simulink library "PC_Simulator_Lib"  (Simulink 8.2)
settings: Solver=ode45  StartTime=0.0  StopTime=10.0  RelTol=1e-3
values from neighbouring files (symbols this model uses):
  data = [r1 r2 r3 r4 L1 L2 L3 L4]    [strasse_Bedatung_HNI_ITI.m]
  distSameLane = 60    [InitialisationsEnv.m]
  eng_speed = [0 60 120 180 240 300 360 420 480 540 600 660 ... (101 elements, 1x101)]    [engine_table.mat]    (also in motor_parameter_calc.m = omega)
  Heading_init = 0    [Start.m]
  inertiaLateral = 25*(radiusWheel)^2    (= 4.129024)    [Start.m]
  laneWidth = 3.6    [InitialisationsEnv.m]    (also in strasse_Bedatung_HNI_ITI.m)
  omega_engine = [0.000000 150.000000 500.000000 1000.000000 1500.000000 2000.000000 2500.000000 3000.000000 3500.000000 4000.000000 4500.000000 5000.000000 5500.000000 6000.000000]    [friction_tables.m]
  omega_max = 6000    [engine_table.mat]    (also in motor_parameter_calc.m)
  omega_wheel = [0 20 40 60 80 100 122 143.7 164]    [friction_tables.m]
  para_Fellow_8_Points = ADAS.Fellow_8_Points    [ADAS_parameters.m]
  position_start_x = [x1 x2 x3 x4 x5 x6 x7]    [strasse_Bedatung_HNI_ITI.m]
  position_start_y = [y1 y2 y3 y4 y5 y6 y7]    [strasse_Bedatung_HNI_ITI.m]
  rad3rdLine = 57.2    [InitialisationsEnv.m]    (also in strasse_Bedatung_HNI_ITI.m)
  radiusWheel = 16*2.54/100    (= 0.4064)    [Start.m]
  s_values = [S1 S2 S3 S4 S5 S6 S7]    [strasse_Bedatung_HNI_ITI.m]
  segmentLimits = [segment1EndThirdLine                   segment2EndThirdLine                   segment3EndThirdLine                   segment4EndThirdLine                   segment5EndThirdLine                   segment6EndThirdLine                   segment7EndThirdLine                   segment8EndThirdLine                   ]    [InitialisationsEnv.m]    (also in strasse_Bedatung_HNI_ITI.m)
  setPosT = [-1.8 -5.4 -1.8 -5.4 -1.8 -5.4 -1.8 -5.4 -1.8 -5.4]    [InitialisationsEnv.m]
  torque = [297.089227105 300.997600937 304.800343044 308.497453426 312.088932082 315.574779014 318.95499422 322.229577701 325.398529457 328.461849487 331.419537793 334.271594373 ... (101 elements, 1x101)]    [engine_table.mat]    (also in motor_parameter_calc.m = g)
  Torque_lost = [0.000000 -8.777780 -15.000000 -26.800000 -29.600000 -32.700000 -35.900000 -39.300000 -42.800000 -46.500000 -50.300000 -54.300000 -58.500000 -62.800000 ]*0.6    [friction_tables.m]
  Torque_lost_wheel = [0.8 0.8 0.75 0.7 0.4 0.3 0.2 0.07 0.07]*0.2    [friction_tables.m]
  X_init = 0    [Start.m]
  Y_init = 1.8    [Start.m]
  Z_init = 0    [Start.m]
undefined symbols (not defined in the file or in its folder): Acc_Pedal, ADAS, Brake_Pedal, Joystick, Newton, Para, Raphson, Standard_Devices, Steering_Wheel_Angle, UDP_Protocol
libraries: simulink x43, rtwinlib x7, dspnetwork x2, simulink_extras x1, vrlib x1
(part 12 of 13)

== matlab function Drive_Train/4_Wheels_drive_train_and_Brake/RL/Fy_calculator ==
  data: lambda input double; Fy output double; alpha input double; V_x input double; Fz input double; mue input double

function Fy = FM_Fy(lambda,alpha,V_x,Fz,mue)
% This block supports an embeddable subset of the MATLAB language.
% See the help menu for details. 
%% Querkraft

kappa=lambda;
a=tan(alpha*pi/180);
%if V_x >=0 
 %   sign=1;
%else
 %   sign=-1;
%end
a_star=tan(alpha*pi/180)*sign(V_x);
F_z=Fz;
%Parameter

p_Cy1=1.193;
p_Ey1=-1.003;
p_Ey2=-0.532;
p_Ey3=-0.083;
p_Ey4=-4.787;
p_Ey5=0;
p_Ky1=14.95;
p_Ky2=2.13;
p_Ky3=-0.028;
p_Ky4=2;
p_Ky5=0;
p_Ky6=2.5;
p_Ky7=0;
p_Hy1=0;
p_Hy2=0;
p_Vy1=0;
p_Vy2=0;
p_Vy3=0;
p_Vy4=0;
r_By1=6.461;
r_By2=4.196;
r_By3=-0.015;
r_Cy1=1.081;
r_Ey1=0;
r_Ey2=0;
r_Hy1=0;
r_Hy2=0;
r_Vy1=0;
r_Vy2=0;
r_Vy3=0;
r_Vy4=0;
r_Vy5=0;
r_Vy6=0;

lambda_ykappa=1;
lambda_Fz0=1;
lambda_Kya=1;
lambda_Cy=1;
lambda_Vy=1;
lambda_muey=1;
lambda_Hy=1;
lambda_Kygamma=1;
lambda_Ey=1;
lambda_Vykappa=1;

% Unter der Annahme, dass die Vertikallast unverändert bleibt:
df_z=0;

%F_z=5500;
%mue=0.7;
chi_0=1;
chi_1=1;
chi_2=1;
chi_3=1;
chi_4=1;

% Annamhe, dass der Sturz bei null bleibt;

gamma=0;

% Berechnung

B_ykappa=(r_By1+r_By3*gamma^2)*cos(atan(r_By2*(a_star-r_By3)))*lambda_ykappa;
C_ykappa=r_Cy1;
E_ykappa=r_Ey1+r_Ey2*df_z;

S_Hykappa=r_Hy1+r_Hy2*df_z;
kappa_S=kappa+S_Hykappa;

G_ykappa0=cos(C_ykappa*atan(B_ykappa*S_Hykappa-E_ykappa*(B_ykappa*S_Hykappa-atan(B_ykappa*S_Hykappa))));
G_ykappa=cos(C_ykappa*atan(B_ykappa*kappa_S-E_ykappa*(B_ykappa*kappa_S-atan(B_ykappa*kappa_S))))/G_ykappa0;
% G_ykappa=cos(C_ykappa*atan(B_ykappa.*kappa_S-E_ykappa*(B_ykappa.*kappa_S-atan(B_ykappa.*kappa_S))))/G_ykappa0;















K_ygamma0=F_z*(p_Ky6+p_Ky7*df_z)*lambda_Kygamma;
S_Vygamma=F_z*(p_Vy3+p_Vy4*df_z)*gamma*lambda_Kygamma*lambda_muey*chi_2;
K_ya=p_Ky1*lambda_Fz0*F_z*sin(p_Ky4*atan(F_z/((p_Ky2+p_Ky5*gamma^2)*lambda_Fz0*F_z)))/(1+p_Ky3*gamma^2)*chi_3*lambda_Kya;
S_Vy=F_z*(p_Vy1+p_Vy2*df_z)*lambda_Vy*lambda_muey*chi_2+S_Vygamma;
S_Hy=(p_Hy1+p_Hy2*df_z)*lambda_Hy+(K_ygamma0*gamma-S_Vygamma)*chi_0/(K_ya+eps)+chi_4-1;

a_y=a+S_Hy;

D_Vykappa=mue*F_z*(r_Vy1+r_Vy2*df_z+r_Vy3*gamma)*cos(atan(r_Vy4*a))*chi_2;
S_Vykappa=D_Vykappa*sin(r_Vy5*atan(r_Vy6*kappa))*lambda_Vykappa;

C_y=p_Cy1*lambda_Cy;
D_y=mue*F_z*chi_2;
B_y=K_ya/(C_y*D_y+eps);
E_y=(p_Ey1+p_Ey2*df_z)*(1+p_Ey5*gamma^2-(p_Ey3+p_Ey4*gamma)*sign(a_y))*lambda_Ey;

F_y0=D_y*sin(C_y*atan(B_y*a_y-E_y*(B_y*a_y-atan(B_y*a_y))))+S_Vy;

F_y=G_ykappa*F_y0+S_Vykappa;

Fy=F_y;

== matlab function Drive_Train/4_Wheels_drive_train_and_Brake/RR/Fx_calculator ==
  data: lambda input double; Fx output double; alpha input double; Fz input double; mue input double
 function Fx = FM_Fx(lambda,alpha,Fz,mue)
% This block supports an embeddable subset of the MATLAB language.
% See the help menu for details. 

%% Längstkraft
kappa=lambda;
a=tan(alpha*pi/180);
F_z=Fz;
% Parameter
p_Cx1=1.685;
p_Ex1=0.344;
p_Ex2=0.095;
p_Ex3=-0.02;
p_Ex4=0;
p_Kx1=21.51;
p_Kx2=-0.163;
p_Kx3=0.245;
p_Hx1=0;
p_Hx2=0;
p_Vx1=0;
p_Vx2=0;
r_Cx1=1.0902;
r_Bx1=12.35;
r_Bx2=-10.77;
r_Bx3=0;
r_Ex1=0;
r_Ex2=0;
r_Hx1=0.007;            %r_Hx1=0.007;
gamma=0;
lambda_xa=1;
lambda_Cx=1;
lambda_Ex=1;
lambda_Hx=1;
lambda_Vx=1;
lambda_Kxkappa=1;
% Unter der Annahme, dass die Vertikallast unverändert bleibt:
df_z=0;

%F_z=5500;
%mue=0.7;
chi_1=1;

% Berechnung:

B_xa=(r_Bx1+r_Bx3*gamma^2)*cos(atan(r_Bx2*kappa))*lambda_xa;
C_xa=r_Cx1;
E_xa=r_Ex1+r_Ex2*df_z;

S_Hxa=r_Hx1;
a_S=a+S_Hxa;

G_xa0=cos(C_xa*atan(B_xa*S_Hxa-E_xa*(B_xa*S_Hxa-atan(B_xa*S_Hxa))));
G_xa=cos(C_xa*atan(B_xa*a_S-E_xa*(B_xa*a_S-atan(B_xa*a_S))))/G_xa0;

K_xkappa=F_z*(p_Kx1+p_Kx2*df_z)*exp(p_Kx3*df_z)*lambda_Kxkappa;
C_x=p_Cx1*lambda_Cx;
D_x=mue*F_z*chi_1;
B_x=K_xkappa/(C_x*D_x+eps);
E_x=(p_Ex1+p_Ex2*df_z+p_Ex3*df_z^2)*(1-p_Ex4*sign(kappa))*lambda_Ex;

S_Vx=F_z*(p_Vx1+p_Vx2*df_z)*lambda_Vx*lambda_Hx*chi_1;
S_Hx=(p_Hx1+p_Hx2*df_z)*lambda_Hx;
kappa_x=kappa+S_Hx;

F_x0 = D_x*sin(C_x*atan(B_x*kappa_x-E_x*(B_x*kappa_x-atan(B_x*kappa_x))))+S_Vx;
% F_x0 = D_x*sin(C_x*atan(B_x*kappa_x-E_x.*(B_x*kappa_x-atan(B_x*kappa_x))))+S_Vx;
F_x = G_xa*F_x0;
% if F_x>249;
%     F_x=249;
% end
Fx=F_x;

== matlab function Drive_Train/4_Wheels_drive_train_and_Brake/RR/Fy_calculator ==
  data: lambda input double; Fy output double; alpha input double; V_x input double; Fz input double; mue input double

function Fy = FM_Fy(lambda,alpha,V_x,Fz,mue)
% This block supports an embeddable subset of the MATLAB language.
% See the help menu for details. 
%% Querkraft

kappa=lambda;
a=tan(alpha*pi/180);
%if V_x >=0 
 %   sign=1;
%else
 %   sign=-1;
%end
a_star=tan(alpha*pi/180)*sign(V_x);
F_z=Fz;
%Parameter

p_Cy1=1.193;
p_Ey1=-1.003;
p_Ey2=-0.532;
p_Ey3=-0.083;
p_Ey4=-4.787;
p_Ey5=0;
p_Ky1=14.95;
p_Ky2=2.13;
p_Ky3=-0.028;
p_Ky4=2;
p_Ky5=0;
p_Ky6=2.5;
p_Ky7=0;
p_Hy1=0;
p_Hy2=0;
p_Vy1=0;
p_Vy2=0;
p_Vy3=0;
p_Vy4=0;
r_By1=6.461;
r_By2=4.196;
r_By3=-0.015;
r_Cy1=1.081;
r_Ey1=0;
r_Ey2=0;
r_Hy1=0;
r_Hy2=0;
r_Vy1=0;
r_Vy2=0;
r_Vy3=0;
r_Vy4=0;
r_Vy5=0;
r_Vy6=0;

lambda_ykappa=1;
lambda_Fz0=1;
lambda_Kya=1;
lambda_Cy=1;
lambda_Vy=1;
lambda_muey=1;
lambda_Hy=1;
lambda_Kygamma=1;
lambda_Ey=1;
lambda_Vykappa=1;

% Unter der Annahme, dass die Vertikallast unverändert bleibt:
df_z=0;

%F_z=5500;
%mue=0.7;
chi_0=1;
chi_1=1;
chi_2=1;
chi_3=1;
chi_4=1;

% Annamhe, dass der Sturz bei null bleibt;

gamma=0;

% Berechnung

B_ykappa=(r_By1+r_By3*gamma^2)*cos(atan(r_By2*(a_star-r_By3)))*lambda_ykappa;
C_ykappa=r_Cy1;
E_ykappa=r_Ey1+r_Ey2*df_z;

S_Hykappa=r_Hy1+r_Hy2*df_z;
kappa_S=kappa+S_Hykappa;

G_ykappa0=cos(C_ykappa*atan(B_ykappa*S_Hykappa-E_ykappa*(B_ykappa*S_Hykappa-atan(B_ykappa*S_Hykappa))));
G_ykappa=cos(C_ykappa*atan(B_ykappa*kappa_S-E_ykappa*(B_ykappa*kappa_S-atan(B_ykappa*kappa_S))))/G_ykappa0;
% G_ykappa=cos(C_ykappa*atan(B_ykappa.*kappa_S-E_ykappa*(B_ykappa.*kappa_S-atan(B_ykappa.*kappa_S))))/G_ykappa0;















K_ygamma0=F_z*(p_Ky6+p_Ky7*df_z)*lambda_Kygamma;
S_Vygamma=F_z*(p_Vy3+p_Vy4*df_z)*gamma*lambda_Kygamma*lambda_muey*chi_2;
K_ya=p_Ky1*lambda_Fz0*F_z*sin(p_Ky4*atan(F_z/((p_Ky2+p_Ky5*gamma^2)*lambda_Fz0*F_z)))/(1+p_Ky3*gamma^2)*chi_3*lambda_Kya;
S_Vy=F_z*(p_Vy1+p_Vy2*df_z)*lambda_Vy*lambda_muey*chi_2+S_Vygamma;
S_Hy=(p_Hy1+p_Hy2*df_z)*lambda_Hy+(K_ygamma0*gamma-S_Vygamma)*chi_0/(K_ya+eps)+chi_4-1;

a_y=a+S_Hy;

D_Vykappa=mue*F_z*(r_Vy1+r_Vy2*df_z+r_Vy3*gamma)*cos(atan(r_Vy4*a))*chi_2;
S_Vykappa=D_Vykappa*sin(r_Vy5*atan(r_Vy6*kappa))*lambda_Vykappa;

C_y=p_Cy1*lambda_Cy;
D_y=mue*F_z*chi_2;
B_y=K_ya/(C_y*D_y+eps);
E_y=(p_Ey1+p_Ey2*df_z)*(1+p_Ey5*gamma^2-(p_Ey3+p_Ey4*gamma)*sign(a_y))*lambda_Ey;

F_y0=D_y*sin(C_y*atan(B_y*a_y-E_y*(B_y*a_y-atan(B_y*a_y))))+S_Vy;

F_y=G_ykappa*F_y0+S_Vykappa;

Fy=F_y;

== matlab function Drive_Train/4_Wheels_drive_train_and_Brake/FR/Fx_calculator ==
  data: lambda input double; Fx output double; alpha input double; Fz input double; mue input double
 function Fx = FM_Fx(lambda,alpha,Fz,mue)
% This block supports an embeddable subset of the MATLAB language.
% See the help menu for details. 

%% Längstkraft
kappa=lambda;
a=tan(alpha*pi/180);
F_z=Fz;
% Parameter
p_Cx1=1.685;
p_Ex1=0.344;
p_Ex2=0.095;
p_Ex3=-0.02;
p_Ex4=0;
p_Kx1=21.51;
p_Kx2=-0.163;
p_Kx3=0.245;
p_Hx1=0;
p_Hx2=0;
p_Vx1=0;
p_Vx2=0;
r_Cx1=1.0902;
r_Bx1=12.35;
r_Bx2=-10.77;
r_Bx3=0;
r_Ex1=0;
r_Ex2=0;
r_Hx1=0.007;            %r_Hx1=0.007;
gamma=0;
lambda_xa=1;
lambda_Cx=1;
lambda_Ex=1;
lambda_Hx=1;
lambda_Vx=1;
lambda_Kxkappa=1;
% Unter der Annahme, dass die Vertikallast unverändert bleibt:
df_z=0;

%F_z=5500;
%mue=0.7;
chi_1=1;

% Berechnung:

B_xa=(r_Bx1+r_Bx3*gamma^2)*cos(atan(r_Bx2*kappa))*lambda_xa;
C_xa=r_Cx1;
E_xa=r_Ex1+r_Ex2*df_z;

S_Hxa=r_Hx1;
a_S=a+S_Hxa;

G_xa0=cos(C_xa*atan(B_xa*S_Hxa-E_xa*(B_xa*S_Hxa-atan(B_xa*S_Hxa))));
G_xa=cos(C_xa*atan(B_xa*a_S-E_xa*(B_xa*a_S-atan(B_xa*a_S))))/G_xa0;

K_xkappa=F_z*(p_Kx1+p_Kx2*df_z)*exp(p_Kx3*df_z)*lambda_Kxkappa;
C_x=p_Cx1*lambda_Cx;
D_x=mue*F_z*chi_1;
B_x=K_xkappa/(C_x*D_x+eps);
E_x=(p_Ex1+p_Ex2*df_z+p_Ex3*df_z^2)*(1-p_Ex4*sign(kappa))*lambda_Ex;

S_Vx=F_z*(p_Vx1+p_Vx2*df_z)*lambda_Vx*lambda_Hx*chi_1;
S_Hx=(p_Hx1+p_Hx2*df_z)*lambda_Hx;
kappa_x=kappa+S_Hx;

F_x0 = D_x*sin(C_x*atan(B_x*kappa_x-E_x*(B_x*kappa_x-atan(B_x*kappa_x))))+S_Vx;
% F_x0 = D_x*sin(C_x*atan(B_x*kappa_x-E_x.*(B_x*kappa_x-atan(B_x*kappa_x))))+S_Vx;
F_x = G_xa*F_x0;
% if F_x>249;
%     F_x=249;
% end
Fx=F_x;

== matlab function Drive_Train/4_Wheels_drive_train_and_Brake/FR/Fy_calculator ==
  data: lambda input double; Fy output double; alpha input double; V_x input double; Fz input double; mue input double

function Fy = FM_Fy(lambda,alpha,V_x,Fz,mue)
% This block supports an embeddable subset of the MATLAB language.
% See the help menu for details. 
%% Querkraft

kappa=lambda;
a=tan(alpha*pi/180);
%if V_x >=0 
 %   sign=1;
%else
 %   sign=-1;
%end
a_star=tan(alpha*pi/180)*sign(V_x);
F_z=Fz;
%Parameter

p_Cy1=1.193;
p_Ey1=-1.003;
p_Ey2=-0.532;
p_Ey3=-0.083;
p_Ey4=-4.787;
p_Ey5=0;
p_Ky1=14.95;
p_Ky2=2.13;
p_Ky3=-0.028;
p_Ky4=2;
p_Ky5=0;
p_Ky6=2.5;
p_Ky7=0;
p_Hy1=0;
p_Hy2=0;
p_Vy1=0;
p_Vy2=0;
p_Vy3=0;
p_Vy4=0;
r_By1=6.461;
r_By2=4.196;
r_By3=-0.015;
r_Cy1=1.081;
r_Ey1=0;
r_Ey2=0;
r_Hy1=0;
r_Hy2=0;
r_Vy1=0;
r_Vy2=0;
r_Vy3=0;
r_Vy4=0;
r_Vy5=0;
r_Vy6=0;

lambda_ykappa=1;
lambda_Fz0=1;
lambda_Kya=1;
lambda_Cy=1;
lambda_Vy=1;
lambda_muey=1;
lambda_Hy=1;
lambda_Kygamma=1;
lambda_Ey=1;
lambda_Vykappa=1;

% Unter der Annahme, dass die Vertikallast unverändert bleibt:
df_z=0;

%F_z=5500;
%mue=0.7;
chi_0=1;
chi_1=1;
chi_2=1;
chi_3=1;
chi_4=1;

% Annamhe, dass der Sturz bei null bleibt;

gamma=0;

% Berechnung

B_ykappa=(r_By1+r_By3*gamma^2)*cos(atan(r_By2*(a_star-r_By3)))*lambda_ykappa;
C_ykappa=r_Cy1;
E_ykappa=r_Ey1+r_Ey2*df_z;

S_Hykappa=r_Hy1+r_Hy2*df_z;
kappa_S=kappa+S_Hykappa;

G_ykappa0=cos(C_ykappa*atan(B_ykappa*S_Hykappa-E_ykappa*(B_ykappa*S_Hykappa-atan(B_ykappa*S_Hykappa))));
G_ykappa=cos(C_ykappa*atan(B_ykappa*kappa_S-E_ykappa*(B_ykappa*kappa_S-atan(B_ykappa*kappa_S))))/G_ykappa0;
% G_ykappa=cos(C_ykappa*atan(B_ykappa.*kappa_S-E_ykappa*(B_ykappa.*kappa_S-atan(B_ykappa.*kappa_S))))/G_ykappa0;















K_ygamma0=F_z*(p_Ky6+p_Ky7*df_z)*lambda_Kygamma;
S_Vygamma=F_z*(p_Vy3+p_Vy4*df_z)*gamma*lambda_Kygamma*lambda_muey*chi_2;
K_ya=p_Ky1*lambda_Fz0*F_z*sin(p_Ky4*atan(F_z/((p_Ky2+p_Ky5*gamma^2)*lambda_Fz0*F_z)))/(1+p_Ky3*gamma^2)*chi_3*lambda_Kya;
S_Vy=F_z*(p_Vy1+p_Vy2*df_z)*lambda_Vy*lambda_muey*chi_2+S_Vygamma;
S_Hy=(p_Hy1+p_Hy2*df_z)*lambda_Hy+(K_ygamma0*gamma-S_Vygamma)*chi_0/(K_ya+eps)+chi_4-1;

a_y=a+S_Hy;

D_Vykappa=mue*F_z*(r_Vy1+r_Vy2*df_z+r_Vy3*gamma)*cos(atan(r_Vy4*a))*chi_2;
S_Vykappa=D_Vykappa*sin(r_Vy5*atan(r_Vy6*kappa))*lambda_Vykappa;

C_y=p_Cy1*lambda_Cy;
D_y=mue*F_z*chi_2;
B_y=K_ya/(C_y*D_y+eps);
E_y=(p_Ey1+p_Ey2*df_z)*(1+p_Ey5*gamma^2-(p_Ey3+p_Ey4*gamma)*sign(a_y))*lambda_Ey;

F_y0=D_y*sin(C_y*atan(B_y*a_y-E_y*(B_y*a_y-atan(B_y*a_y))))+S_Vy;

F_y=G_ykappa*F_y0+S_Vykappa;

Fy=F_y;

== matlab function ADAS/Sensors_ADAS/Front_Long_Range_Radar_Sensor/First_STage_Coordinate_Transformation/Radar_Triangles_Transformation_From_Local2Global/Coord_Transformatin_Rotation1 ==
  data: roll input double; Trans_Local2Global output double; pitch input double; yaw input double
function Trans_Local2Global  = fcn(roll, pitch, yaw)


Trans_Local2Global=[ cos(pitch)*cos(yaw) cos(yaw)*sin(pitch)*sin(roll) - cos(roll)*sin(yaw) sin(roll)*sin(yaw) + cos(roll)*cos(yaw)*sin(pitch);
cos(pitch)*sin(yaw) cos(roll)*cos(yaw) + sin(pitch)*sin(roll)*sin(yaw) cos(roll)*sin(pitch)*sin(yaw) - cos(yaw)*sin(roll);
         -sin(pitch)                               cos(pitch)*sin(roll)                               cos(pitch)*cos(roll)];

== matlab function ADAS/Decision_Making_ADAS/Trajectory_calculatin_and_distance_control_and output_maping/Calculate_Desired_Trajectory/Road model ST_XY/st_xy ==
  data: x output double; s input double; t input double; y output double; z output double; headingAngle output double; curvature output double; friction output double; segmentNr output double; segmentLimits input double; laneWidth input double; rad3rdLine input double
function [x, y, z, headingAngle, curvature, friction, segmentNr]   = st_xy(s, t, segmentLimits, laneWidth, rad3rdLine)
%% Description
% This function transforms the (s,t) points of the road to (x,y) points
% From local coordinate system to global coordinate system
% s,t: s,t points of the local coordinate system in meters
% segmentLimits: Limits, i.e. ends, of road segments in meters
% laneWidth: The width of the lane in meter
% rad3rdLine: Radius of the third line, i.e lane marking, in meter  
% x,y: x,y points of the global coordinate system in meters
% headingAngle: Heading angle of the road at a specific road segment
% curvature: Curvature of the road at a specific road segment
% segmentNr: Segment number of a specific (s,t) point on the road
%% Simple schematic for a slice of the road
%     |          |         |          |          |
% FirstLine SecondLine ThirdLine FourthLine FifthLine 
%        Lane 2     Lane 1    Lane -1    Lane -2
%% Simple schematic for the road shape
%  _____________________
% (                     )
% |                     |
% |                     |
% |                     |
% (_____________________)

%% Initialise the outputs (Assign default values)
% Initialise x with zero
x = 0; 
% Initialise y with zero
y = 0;
% Initialise z with zero
z = 0;
% Initialise segmentNr with zero
segmentNr = 0;
% Initialise headingAngle with zero
headingAngle = 0;
% Initialise curvature with zero
curvature = 0;
% Initialise friction coefficient (Asphalt)
friction = 0.72;

%% Check (s,t) point against all segments
%% Check if the point is in the 1st road segment (Straight line)
if(s>=0)&&(s<segmentLimits(1))  
    % Calculate x component
    x = s;
    % Calculate y component
    y = t;
    % Calculate z value
    z = 0;
    % Calculate heading angle
    headingAngle = 0;
    % Calculate curvature
    curvature = 0;
    % Set friction value
    friction  = 0.72;
    % Set segment number
    segmentNr = 1;
%% Check if the point is in the 2nd road segment
elseif(s>=segmentLimits(1)) && (s<segmentLimits(2)) 
    % Calculate x component
    x = (rad3rdLine-t)*sin((s-segmentLimits(1))/rad3rdLine) + 600;
    % Calculate y component
    y = rad3rdLine - (rad3rdLine-t)*cos((s-segmentLimits(1))/rad3rdLine);
    % Calculate z value
    z = 0;
    % Calculate heading angle
    headingAngle = (180/pi)*(s-600)/rad3rdLine;
    % Calculate curvature
    curvature = 1/(rad3rdLine-t);
    % Set friction value
    friction  = 0.72;
    % Set segment number
    segmentNr = 2;
%% Check if the point is in the 3rd road segment  
elseif(s>=segmentLimits(2)) && (s<segmentLimits(3))
    % Calculate x component
    x = -t + 600 + rad3rdLine;
    % Calculate y component
    y = (s-segmentLimits(2)) + rad3rdLine;
    % Calculate z value
    z = 0;
    % Calculate heading angle
    headingAngle = 90;
    % Calculate curvature
    curvature = 0;
    % Set friction value
    friction  = 0.72;
    % Set segment number
    segmentNr = 3;
%% Check if the point is in the 4th road segment
elseif(s>=segmentLimits(3)) && (s<segmentLimits(4))
    % Calculate x component
    x = (rad3rdLine-t)*cos((s-segmentLimits(3))/rad3rdLine) - rad3rdLine + 600 + rad3rdLine;
    % Calculate y component
    y = (rad3rdLine-t)*sin((s-segmentLimits(3))/rad3rdLine) + 300 + rad3rdLine;
    % Calculate z value
    z = 0;
    % Calculate heading angle
    headingAngle = ((180/pi)*(s-(600+89.8857+300))/rad3rdLine) + 90;
    % Calculate curvature
    curvature = 1/(rad3rdLine-t);
    % Set friction value
    friction  = 0.72;
    % Set segment number
    segmentNr = 4;
%% Check if the point is in the 5th road segment
elseif(s>=segmentLimits(4))&&(s<segmentLimits(5))
    % Calculate x component
    x = -(s-segmentLimits(4)) + 600;
    % Calculate y component
    y = -t + (4*laneWidth) + 50 + 300 + 50;
    % Calculate z value
    z = 0;
    % Calculate heading angle
    headingAngle = 180;
    % Calculate curvature
    curvature = 0;
    % Set friction value
    friction  = 0.72;
    % Set segment number
    segmentNr = 5;
%% Check if the point is in the 6th road segment  
elseif(s>=segmentLimits(5))&&(s<segmentLimits(6))
    % Calculate x component
    x = -(rad3rdLine-t)*sin((s-segmentLimits(5))/rad3rdLine);
    % Calculate y component
    y = (rad3rdLine-t)*cos((s-segmentLimits(5))/rad3rdLine)- rad3rdLine + (4*laneWidth) + 50 + 300 + 50;
    % Calculate z value
    z = 0;
    % Calculate heading angle
    headingAngle = ((180/pi)*(s-(600+89.8857+300+89.8857+600))/rad3rdLine) + 180;
    % Calculate curvature
    curvature = 1/(rad3rdLine-t);
    % Set friction value
    friction  = 0.72;
    % Set segment number
    segmentNr = 6;
%% Check if the point is in the 7th road segment 
elseif(s>=segmentLimits(6))&&(s<segmentLimits(7))
    % Calculate x component
    x = t- 50 - 3.6 - 3.6;
    % Calculate y component
    y = -(s-segmentLimits(6)) + (2*laneWidth) + 300 + 50;
    % Calculate z value
    z = 0;
    % Calculate heading angle
    headingAngle = 270;
    % Calculate curvature
    curvature = 0;
    % Set friction value
    friction  = 0.72;
    % Set segment number
    segmentNr = 7;
%% Check if the point is in the 8th road segment 
elseif(s>=segmentLimits(7))&&(s<segmentLimits(8))
    % Calculate x component
    x = rad3rdLine-(rad3rdLine-t)*cos((s-segmentLimits(7))/rad3rdLine) - rad3rdLine;
    % Calculate y component
    y = -(rad3rdLine-t)*sin((s-segmentLimits(7))/rad3rdLine) + rad3rdLine; 
    % Calculate z value
    z = 0;
    % Calculate heading angle
    headingAngle = ((180/pi)*(s-(600+89.8857+300+89.8857+600+89.8857+300))/rad3rdLine) + 270;
    % Calculate curvature
    curvature = 1/(rad3rdLine-t);
    % Set friction value
    friction  = 0.72;
    % Set segment number
    segmentNr = 8;
end
end

== matlab function ADAS/Decision_Making_ADAS/Trajectory_calculatin_and_distance_control_and output_maping/Calculate_Desired_Trajectory/Strasse_xy/Embedded MATLAB Function ==
  data: data input double; position_start_x input double; position_start_y input double; s_values input double; x input double; y input double; z output double; psi output double; mue output double; s output double; t output double
function [z,psi,mue,s,t] = fcn(data,position_start_x,position_start_y,s_values,x,y)


breite=14.4;
margin=3;

if x>=0 && x<position_start_x(1) && y>=-(breite/2+margin) && y<=(breite/2+margin)                                               %S1
    s=x;
    t=y;
    psi=0;
else if x>=position_start_x(1) && x<(position_start_x(2)+breite/2+margin) && y>=-(breite/2+margin) && y<=position_start_y(2)    %S2
        phi=atan((x-position_start_x(1))/(position_start_y(2)-y));
        r=sqrt((x-position_start_x(1))^2 + (position_start_y(2)-y)^2);
        s=data(1)*phi+s_values(1);
        t=data(1)-r;
        psi=phi;
        
else if x>=(position_start_x(2)-breite/2-margin) && x<=(position_start_x(2)+breite/2+margin) && y>position_start_y(2) && y<position_start_y(3)  %S3
        s=s_values(2)+(y-position_start_y(2));
        t=position_start_x(2)-x;
        psi=pi/2;
        
else if  x<=(position_start_x(3)+breite/2+margin) && x>=(position_start_x(4)) && y>=position_start_y(3) && y<=(position_start_y(4)+breite/2+margin)   %S4
        phi=atan((y-position_start_y(3))/(x-position_start_x(4)));
        r=sqrt((y-position_start_y(3))^2+(x-position_start_x(4))^2);
        s=s_values(3)+data(2)*phi;
        t=data(2)-r;
        psi=pi/2+phi;
        
else if x<position_start_x(4) && x>position_start_x(5) && y>=(position_start_y(4)-breite/2-margin) && y<(position_start_y(4)+breite/2+margin)   %S5
        s=s_values(4)+(position_start_x(4)-x);
        t=position_start_y(4)-y;
        psi=pi;
        
else if x<=position_start_x(5) && x>=(position_start_x(6)-breite/2-margin) && y>=position_start_y(6) && y<=(position_start_y(5)+breite/2+margin)   %S6
        phi=atan(-x/(y-position_start_y(6)));
        r=sqrt((x)^2+(y-position_start_y(6))^2);
        s=s_values(5)+data(3)*phi;
        t=data(3)-r;
        psi=pi+phi;
        
else if x>=(position_start_x(6)-breite/2-margin) && x<=(position_start_x(6)+breite/2+margin) && y>position_start_y(7) && y<position_start_y(6)   %S7
        s=s_values(6)+(position_start_y(6)-y);
        t=x-position_start_x(6);
        psi=3*pi/2;
        
else if x>=(position_start_x(7)-breite/2-margin) && x<0 && y>=(-breite/2-margin) && y<=position_start_y(7)   %S8
        phi=atan((position_start_y(7)-y)/(-x));
        r=sqrt((position_start_y(7)-y)^2+(x)^2);
        s=s_values(7)+data(4)*phi;
        t=data(4)-r;
        psi=3*pi/2+phi;     
        

     else
         s=0;
         t=0;
         psi=0;

    end
    end
    end
    end
    end
    end
    end
end
    
z=0;
mue=1;

== matlab function ADAS/Sensors_ADAS/Front_Long_Range_Radar_Sensor/Coordinate_TRansformation_of_Fellows_Points_Plus_Calculation_Distances_And_Angles/MATLAB Function ==
  data: Objects_Dectected input double; Position_Fellows input double; Oriantation_Fellows input double; Apex_Pos_Global input double; yaw_VUT input double; delta_s output double; Angle output double; para_num_fellow parameter double; para_Fellow_8_Points parameter double; position output double
function [delta_s,Angle,position] = fcn(Objects_Dectected,Position_Fellows,Oriantation_Fellows,Apex_Pos_Global,yaw_VUT,para_num_fellow,para_Fellow_8_Points)
%%
Fellow_Points=zeros(para_num_fellow,24);
delta_distance=zeros(para_num_fellow,2);
Angles_Array=zeros(para_num_fellow,1);
position_Array=zeros(para_num_fellow,3,2);
% index=-1; %only for testing

% pass inputs and calculate the transformation matrix 
for i=0:para_num_fellow-1
    if Objects_Dectected(i+1)==1
    roll=Oriantation_Fellows(i*3+1);
    pitch=Oriantation_Fellows(i*3+2);
    yaw=Oriantation_Fellows(i*3+3);
    Trans_Local2Global=[ cos(pitch)*cos(yaw) cos(yaw)*sin(pitch)*sin(roll) - cos(roll)*sin(yaw) sin(roll)*sin(yaw) + cos(roll)*cos(yaw)*sin(pitch);
    cos(pitch)*sin(yaw) cos(roll)*cos(yaw) + sin(pitch)*sin(roll)*sin(yaw) cos(roll)*sin(pitch)*sin(yaw) - cos(yaw)*sin(roll);
         -sin(pitch)                               cos(pitch)*sin(roll)                               cos(pitch)*cos(roll)];
     
     FLU=Trans_Local2Global*para_Fellow_8_Points.FLU+[Position_Fellows(i*3+1);Position_Fellows(i*3+2);Position_Fellows(i*3+3)];
     FLL=Trans_Local2Global*para_Fellow_8_Points.FLL+[Position_Fellows(i*3+1);Position_Fellows(i*3+2);Position_Fellows(i*3+3)];
     FRU=Trans_Local2Global*para_Fellow_8_Points.FRU+[Position_Fellows(i*3+1);Position_Fellows(i*3+2);Position_Fellows(i*3+3)];
     FRL=Trans_Local2Global*para_Fellow_8_Points.FRL+[Position_Fellows(i*3+1);Position_Fellows(i*3+2);Position_Fellows(i*3+3)];
     RLU=Trans_Local2Global*para_Fellow_8_Points.RLU+[Position_Fellows(i*3+1);Position_Fellows(i*3+2);Position_Fellows(i*3+3)];
     RLL=Trans_Local2Global*para_Fellow_8_Points.RLL+[Position_Fellows(i*3+1);Position_Fellows(i*3+2);Position_Fellows(i*3+3)];
     RRU=Trans_Local2Global*para_Fellow_8_Points.RRU+[Position_Fellows(i*3+1);Position_Fellows(i*3+2);Position_Fellows(i*3+3)];
     RRL=Trans_Local2Global*para_Fellow_8_Points.RRL+[Position_Fellows(i*3+1);Position_Fellows(i*3+2);Position_Fellows(i*3+3)];
     A=[FLU ; FLL ; FRU ; FRL ; RLU ; RLL ; RRU ; RRL];
     Fellow_Points(i+1,:)=A;  %what is that
     dist1=sqrt(sum((Apex_Pos_Global-FLU).^2));
     dist2=sqrt(sum((Apex_Pos_Global-FLL).^2));
     dist3=sqrt(sum((Apex_Pos_Global-FRU).^2));
     dist4=sqrt(sum((Apex_Pos_Global-FRL).^2));
     dist5=sqrt(sum((Apex_Pos_Global-RLU).^2));
     dist6=sqrt(sum((Apex_Pos_Global-RLL).^2));
     dist7=sqrt(sum((Apex_Pos_Global-RRU).^2));
     dist8=sqrt(sum((Apex_Pos_Global-RRL).^2));     
     
     Dist=[dist1 dist2 dist3 dist4 dist5 dist6 dist7 dist8];
     [~, index_Sort_Arr]=sort(Dist);
     Angle1=abs((atan2((A((index_Sort_Arr(1)-1)*3+2)-Apex_Pos_Global(2)),(A((index_Sort_Arr(1)-1)*3+1)-Apex_Pos_Global(1))))-yaw_VUT);
     Angle2=abs((atan2((A((index_Sort_Arr(2)-1)*3+2)-Apex_Pos_Global(2)),(A((index_Sort_Arr(2)-1)*3+1)-Apex_Pos_Global(1))))-yaw_VUT);
     Angle3=abs((atan2((A((index_Sort_Arr(3)-1)*3+2)-Apex_Pos_Global(2)),(A((index_Sort_Arr(3)-1)*3+1)-Apex_Pos_Global(1))))-yaw_VUT);
     [~,index_angle_min]=min([Angle1 Angle2 Angle3]);
     [~,index_angle_max]=max([Angle1 Angle2 Angle3]);
     index_min=index_Sort_Arr(index_angle_min);
     index_max=index_Sort_Arr(index_angle_max);     
%      [delta_distance(i+1), index]=min([dist1 dist2 dist3 dist4 dist5 dist6 dist7 dist8]);
     delta_distance(i+1,1)=Dist(index_min);
     delta_distance(i+1,2)=Dist(index_max);
%      Angles_Array(i+1)=(atan2((A((index-1)*3+2)-Apex_Pos_Global(2)),(A((index-1)*3+1)-Apex_Pos_Global(1))))-yaw_VUT;
%      position_Array(i+1,:)=[A((index-1)*3+1) A((index-1)*3+2) A((index-1)*3+3)];
     position_Array(i+1,:,1)=[A((index_min-1)*3+1) A((index_min-1)*3+2) A((index_min-1)*3+3)];
     position_Array(i+1,:,2)=[A((index_max-1)*3+1) A((index_max-1)*3+2) A((index_max-1)*3+3)];
    end
end
%%
%pass the output

delta_s=delta_distance;
Angle=Angles_Array;
position=position_Array;

== matlab function ADAS/Sensors_ADAS/Front_Mid_Range_Radar_Sensor/First_STage_Coordinate_Transformation/Radar_Triangles_Transformation_From_Local2Global/Coord_Transformatin_Rotation1 ==
  data: roll input double; Trans_Local2Global output double; pitch input double; yaw input double
function Trans_Local2Global  = fcn(roll, pitch, yaw)


Trans_Local2Global=[ cos(pitch)*cos(yaw) cos(yaw)*sin(pitch)*sin(roll) - cos(roll)*sin(yaw) sin(roll)*sin(yaw) + cos(roll)*cos(yaw)*sin(pitch);
cos(pitch)*sin(yaw) cos(roll)*cos(yaw) + sin(pitch)*sin(roll)*sin(yaw) cos(roll)*sin(pitch)*sin(yaw) - cos(yaw)*sin(roll);
         -sin(pitch)                               cos(pitch)*sin(roll)                               cos(pitch)*cos(roll)];

== stateflow chart ADAS/Unser_Interface_ADAS/ACC_User_Interface/ACC_User_Control ==
  state ActiveSet
    en:
    Set_Speed=Velocity_VUT;
    Last_Set_Speed=Velocity_VUT;
    ACC_State=1;
    First_Set=0;
    state Default
    state Plus
      en:
      Last_Set_Speed=min(Last_Set_Speed+5/3.6, 200/3.6);
      Set_Speed=Last_Set_Speed;
    state Minus
      Last_Set_Speed=max(Last_Set_Speed-5/3.6,0);
      Set_Speed=Last_Set_Speed;
    (default) -> Default
    Default -> Plus [order 1] : Button_Plus
    Default -> Minus [order 2] : Button_Minus
    Minus -> Default
    Plus -> Default
  state ActiveResume
    en:
    Set_Speed=Last_Set_Speed;
    ACC_State=1;
    state Default1
    state Minus1
      Last_Set_Speed=max(Last_Set_Speed-5/3.6,0);
      Set_Speed=Last_Set_Speed;
    state Plus1
      en:
      Last_Set_Speed=min(Last_Set_Speed+5/3.6, 200/3.6);
      Set_Speed=Last_Set_Speed;
    (default) -> Default1
    Default1 -> Plus1 [order 1] : Button_Plus
    Default1 -> Minus1 [order 2] : Button_Minus
    Minus1 -> Default1
    Plus1 -> Default1
  state Standby
    ACC_State=0;
  state Standby1
    ACC_State=0;
  Standby1 -> ActiveResume [order 1] : [Gas_Pedal_User<=Gas_Pedal_ACC]
  Standby -> ActiveResume [order 2] : Button_Resume[Gearbox_State==1 && First_Set==0 && Enabled_Systems==0]
  Standby -> ActiveSet [order 1] : Button_Plus || Button_Minus   [Gearbox_State==1 && Enabled_Systems==0 ]
  ActiveSet -> Standby [order 2] : [ Gearbox_State!=1 || Brake_Pedal_User>Brake_Pedal_ACC ]
  ActiveSet -> Standby [order 1] : Button_Stop
  ActiveSet -> Standby1 [order 3] : [Gas_Pedal_User>Gas_Pedal_ACC]
  ActiveResume -> Standby1 [order 3] : [Gas_Pedal_User>Gas_Pedal_ACC]
  ActiveResume -> Standby [order 1] : Button_Stop
  ActiveResume -> Standby [order 2] : [ Gearbox_State!=1 || Brake_Pedal_User>Brake_Pedal_ACC ]
  (default) -> Standby
  Standby1 -> Standby [order 2] : Button_Stop
  Standby1 -> Standby [order 3] : [ Gearbox_State!=1 || Brake_Pedal_User>Brake_Pedal_ACC ]
  data: ACC_State output double =0; Gearbox_State input double; Gas_Pedal_User input double; Brake_Pedal_User input double; Velocity_VUT input double; Gas_Pedal_ACC input double; Brake_Pedal_ACC input double; Set_Speed output double =0; Last_Set_Speed local double =0; First_Set local double =1; Enabled_Systems input double
  events: update input EITHER_EDGE_EVENT; Button_Plus input RISING_EDGE_EVENT; Button_Minus input RISING_EDGE_EVENT; Button_Stop input RISING_EDGE_EVENT; Button_Resume input RISING_EDGE_EVENT

== stateflow chart ADAS/Unser_Interface_ADAS/ACC_User_Interface/Time_Gap_switching ==
  state Sporty
    en:
    Time_Gap=1;
  state Comfortable
    en:
    Time_Gap=2.3;
  state SemiComfortable
    en:
    Time_Gap=1.8;
  state SemiSporty
    en:
    Time_Gap=1.3;
  note: the values and the modes
      | are from the Audi A8 Prese
  Sporty -> SemiSporty : Button
  Comfortable -> Sporty : Button
  SemiSporty -> SemiComfortable : Button
  SemiComfortable -> Comfortable : Button
  (default) -> Comfortable
  data: Time_Gap output double
  events: Update input EITHER_EDGE_EVENT; Button input RISING_EDGE_EVENT

== stateflow chart ADAS/Unser_Interface_ADAS/Emergency_Brake/Emergency_brake_HMI_model ==
  state On
    en:
    State=1;
  state Off
    en:
    State=0;
  On -> Off : Button
  Off -> On : Button[Enabled_Systems==0]
  (default) -> Off
  data: State output double; Enabled_Systems input double
  events: Update input EITHER_EDGE_EVENT; Button input RISING_EDGE_EVENT

== matlab function ADAS/Sensors_ADAS/Front_Mid_Range_Radar_Sensor/Coordinate_TRansformation_of_Fellows_Points_Plus_Calculation_Distances_And_Angles/MATLAB Function ==
  data: Objects_Dectected input double; Position_Fellows input double; Oriantation_Fellows input double; Apex_Pos_Global input double; yaw_VUT input double; delta_s output double; Angle output double; para_num_fellow parameter double; para_Fellow_8_Points parameter double; position output double
function [delta_s,Angle,position] = fcn(Objects_Dectected,Position_Fellows,Oriantation_Fellows,Apex_Pos_Global,yaw_VUT,para_num_fellow,para_Fellow_8_Points)
%%
Fellow_Points=zeros(para_num_fellow,24);
delta_distance=zeros(para_num_fellow,2);
Angles_Array=zeros(para_num_fellow,1);
position_Array=zeros(para_num_fellow,3,2);
% index=-1; %only for testing

% pass inputs and calculate the transformation matrix 
for i=0:para_num_fellow-1
    if Objects_Dectected(i+1)==1
    roll=Oriantation_Fellows(i*3+1);
    pitch=Oriantation_Fellows(i*3+2);
    yaw=Oriantation_Fellows(i*3+3);
    Trans_Local2Global=[ cos(pitch)*cos(yaw) cos(yaw)*sin(pitch)*sin(roll) - cos(roll)*sin(yaw) sin(roll)*sin(yaw) + cos(roll)*cos(yaw)*sin(pitch);
    cos(pitch)*sin(yaw) cos(roll)*cos(yaw) + sin(pitch)*sin(roll)*sin(yaw) cos(roll)*sin(pitch)*sin(yaw) - cos(yaw)*sin(roll);
         -sin(pitch)                               cos(pitch)*sin(roll)                               cos(pitch)*cos(roll)];
     
     FLU=Trans_Local2Global*para_Fellow_8_Points.FLU+[Position_Fellows(i*3+1);Position_Fellows(i*3+2);Position_Fellows(i*3+3)];
     FLL=Trans_Local2Global*para_Fellow_8_Points.FLL+[Position_Fellows(i*3+1);Position_Fellows(i*3+2);Position_Fellows(i*3+3)];
     FRU=Trans_Local2Global*para_Fellow_8_Points.FRU+[Position_Fellows(i*3+1);Position_Fellows(i*3+2);Position_Fellows(i*3+3)];
     FRL=Trans_Local2Global*para_Fellow_8_Points.FRL+[Position_Fellows(i*3+1);Position_Fellows(i*3+2);Position_Fellows(i*3+3)];
     RLU=Trans_Local2Global*para_Fellow_8_Points.RLU+[Position_Fellows(i*3+1);Position_Fellows(i*3+2);Position_Fellows(i*3+3)];
     RLL=Trans_Local2Global*para_Fellow_8_Points.RLL+[Position_Fellows(i*3+1);Position_Fellows(i*3+2);Position_Fellows(i*3+3)];
     RRU=Trans_Local2Global*para_Fellow_8_Points.RRU+[Position_Fellows(i*3+1);Position_Fellows(i*3+2);Position_Fellows(i*3+3)];
     RRL=Trans_Local2Global*para_Fellow_8_Points.RRL+[Position_Fellows(i*3+1);Position_Fellows(i*3+2);Position_Fellows(i*3+3)];
     A=[FLU ; FLL ; FRU ; FRL ; RLU ; RLL ; RRU ; RRL];
     Fellow_Points(i+1,:)=A;  %what is that
     dist1=sqrt(sum((Apex_Pos_Global-FLU).^2));
     dist2=sqrt(sum((Apex_Pos_Global-FLL).^2));
     dist3=sqrt(sum((Apex_Pos_Global-FRU).^2));
     dist4=sqrt(sum((Apex_Pos_Global-FRL).^2));
     dist5=sqrt(sum((Apex_Pos_Global-RLU).^2));
     dist6=sqrt(sum((Apex_Pos_Global-RLL).^2));
     dist7=sqrt(sum((Apex_Pos_Global-RRU).^2));
     dist8=sqrt(sum((Apex_Pos_Global-RRL).^2));     
     
     Dist=[dist1 dist2 dist3 dist4 dist5 dist6 dist7 dist8];
     [~, index_Sort_Arr]=sort(Dist);
     Angle1=abs((atan2((A((index_Sort_Arr(1)-1)*3+2)-Apex_Pos_Global(2)),(A((index_Sort_Arr(1)-1)*3+1)-Apex_Pos_Global(1))))-yaw_VUT);
     Angle2=abs((atan2((A((index_Sort_Arr(2)-1)*3+2)-Apex_Pos_Global(2)),(A((index_Sort_Arr(2)-1)*3+1)-Apex_Pos_Global(1))))-yaw_VUT);
     Angle3=abs((atan2((A((index_Sort_Arr(3)-1)*3+2)-Apex_Pos_Global(2)),(A((index_Sort_Arr(3)-1)*3+1)-Apex_Pos_Global(1))))-yaw_VUT);
     [~,index_angle_min]=min([Angle1 Angle2 Angle3]);
     [~,index_angle_max]=max([Angle1 Angle2 Angle3]);
     index_min=index_Sort_Arr(index_angle_min);
     index_max=index_Sort_Arr(index_angle_max);     
%      [delta_distance(i+1), index]=min([dist1 dist2 dist3 dist4 dist5 dist6 dist7 dist8]);
     delta_distance(i+1,1)=Dist(index_min);
     delta_distance(i+1,2)=Dist(index_max);
%      Angles_Array(i+1)=(atan2((A((index-1)*3+2)-Apex_Pos_Global(2)),(A((index-1)*3+1)-Apex_Pos_Global(1))))-yaw_VUT;
%      position_Array(i+1,:)=[A((index-1)*3+1) A((index-1)*3+2) A((index-1)*3+3)];
     position_Array(i+1,:,1)=[A((index_min-1)*3+1) A((index_min-1)*3+2) A((index_min-1)*3+3)];
     position_Array(i+1,:,2)=[A((index_max-1)*3+1) A((index_max-1)*3+2) A((index_max-1)*3+3)];
    end
end
%%
%pass the output

delta_s=delta_distance;
Angle=Angles_Array;
position=position_Array;

== matlab function ADAS/Sensors_ADAS/Object_Selection_Based_On_LRR_MRR_and_Camera SENSOR FUSION/MATLAB Function ==
  data: object_in_lane output double; objects_dectected_LRR input double; delta_s_vector_LRR input double; angle_H_vector_LRR input double; distance output double; T_Objects_LRR input double; objects_dectected_MRR input double; delta_s_vector_MRR input double; angle_H_vector_MRR input double; T_Objects_MRR input double; T_VUT input double; direction_delta_T output double; distance_lateral output double
function [object_in_lane, distance,direction_delta_T, distance_lateral] = fcn(objects_dectected_LRR,delta_s_vector_LRR,angle_H_vector_LRR,T_Objects_LRR,objects_dectected_MRR,delta_s_vector_MRR,angle_H_vector_MRR,T_Objects_MRR,T_VUT)
%%
% allocate memory for the matrix used in the code
% the size of the matrix depends on objects that intersect the field of sensor  
objects_detected=objects_dectected_LRR|objects_dectected_MRR;
index_Objects_detected=find(objects_detected==1);
delta_s_vector_ini=zeros(length(index_Objects_detected),2);
T_Objects_ini=zeros(length(index_Objects_detected),2);
angle_H_vector_ini=zeros(length(index_Objects_detected),1);
d_Fellows_min=zeros(length(index_Objects_detected),1);
index_t_min=zeros(length(index_Objects_detected),1);
lateral_dist=zeros(1,2);
%%
%from the objects in the field of sensor the related object is the one to
%be selectin this section
%in this 2 for-loops the pre-alocated matrix will be filled with the data
%from the inputs, the input is represnting the data for all fellow
%vehicles, while here the data of the vehicls in the sensor region only is
%to be tested
for j=1:2
for i=1:length(index_Objects_detected)
    if objects_dectected_LRR(index_Objects_detected(i))==1
        delta_s_vector_ini(i,j)=delta_s_vector_LRR(index_Objects_detected(i),j);    
        angle_H_vector_ini(i)=angle_H_vector_LRR(index_Objects_detected(i));
        T_Objects_ini(i,j)=T_Objects_LRR(index_Objects_detected(i),j); 
    else
        delta_s_vector_ini(i,j)=delta_s_vector_MRR(index_Objects_detected(i),j);    
        angle_H_vector_ini(i)=angle_H_vector_MRR(index_Objects_detected(i));
        T_Objects_ini(i,j)=T_Objects_MRR(index_Objects_detected(i),j);
    end
end
end
%%
% find if one of the objects in on the way of the vehicle under test and
% what is the distance to it
d_Fellows=abs(T_Objects_ini-T_VUT);
for i=1:length(index_Objects_detected)
    [d_Fellows_min(i),index_t_min(i)]=min(d_Fellows(i,:));
end
index_Array=find(d_Fellows_min<=0.9);
index=-1;
dest=1000;
% alpha=0;
for i=1:length(index_Array)
    if delta_s_vector_ini(index_Array(i),index_t_min(index_Array(i)))<dest
        dest=delta_s_vector_ini(index_Array(i),index_t_min(index_Array(i)));
%         alpha=angle_H_vector_ini(index_Array(i));
        index=index_Array(i);
    end
end
%%
% if there is no vehicle on the way of the vehicle
if index==-1
object_in_lane=0;
distance=0;
direction_delta_T=0;
distance_lateral=0;

else
    %%if there is a vehicle on the way of the vehicle
    object_in_lane=1;
%     distance=dest*cos(alpha);
    distance=dest;
    
    %%
    %the investigation of steering chances inside the same
    
    %if the VUT was in the most right lane (4th lane from left)
    if T_VUT>=-7.2  && T_VUT<-3.6                                   
        T_Edges_rel=sort(T_Objects_ini(index,:)+3.6);
        if T_Edges_rel(2)<=0
            lateral_dist(1)=-T_Edges_rel(2);
        else
            lateral_dist(1)=0;
        end
        if T_Edges_rel(1)>=-3.6
            lateral_dist(2)=T_Edges_rel(1)+3.6;
        else
            lateral_dist(2)=0;
        end          
        
        %if the VUT was in the 3rd lane from left
    else if T_VUT>=-3.6  && T_VUT<0                                 
             T_Edges_rel=sort(T_Objects_ini(index,:));
        if T_Edges_rel(2)<=0
            lateral_dist(1)=-T_Edges_rel(2);
        else
            lateral_dist(1)=0;
        end
        if T_Edges_rel(1)>=-3.6
            lateral_dist(2)=T_Edges_rel(1)+3.6;
        else
            lateral_dist(2)=0;
        end      
           %if the VUT was in the 2nd lane from left
        else if T_VUT>=0  && T_VUT<3.6                              
                  T_Edges_rel=sort(T_Objects_ini(index,:));
        if T_Edges_rel(2)<=3.6
            lateral_dist(1)=3.6-T_Edges_rel(2);
        else
            lateral_dist(1)=0;
        end
        if T_Edges_rel(1)>=0
            lateral_dist(2)=T_Edges_rel(1);
        else
            lateral_dist(2)=0;
        end                     
                %if the VUT was in the 2nd lane from left
            else if T_VUT>=3.6  && T_VUT<7.2                        
             T_Edges_rel=sort(T_Objects_ini(index,:)-3.6);
        if T_Edges_rel(2)<=3.6
            lateral_dist(1)=3.6-T_Edges_rel(2);
        else
            lateral_dist(1)=0;
        end
        if T_Edges_rel(1)>=0
            lateral_dist(2)=T_Edges_rel(1);
        else
            lateral_dist(2)=0;
        end        
        %not on the road
                else                                           
                    lateral_dist=[0 0];    
                   
                end
            end
        end        
    end
    T_Edges=sort(T_Objects_ini(index,:));
   if  lateral_dist(1)>=1.5
       direction_delta_T=1;
        distance_lateral=T_Edges(2)-T_VUT;
   else if lateral_dist(2)>=1.5
            direction_delta_T=-1;
            distance_lateral=T_Edges(1)-T_VUT;
       else
            direction_delta_T=0;
            distance_lateral=0;
       end
   end
   
end

== matlab function ADAS/Sensors_ADAS/convert_xy_2_st/Embedded MATLAB Function ==
  data: data input double; position_start_x input double; position_start_y input double; s_values input double; Positon_of_detected_Points input double; z output double; psi output double; mue output double; s output double; t output double; para_num_fellow parameter double
function [z,psi,mue,s,t] = fcn(data,position_start_x,position_start_y,s_values,Positon_of_detected_Points,para_num_fellow)

x=zeros(para_num_fellow,2);
y=zeros(para_num_fellow,2);
t_array=zeros(para_num_fellow,2);
for j=1:2
for i=1:para_num_fellow
    x(i,j)=Positon_of_detected_Points(i,1,j);
    y(i,j)=Positon_of_detected_Points(i,2,j);
end
end
breite=14.4;
margin=5;
for j=1:2
for i=1:para_num_fellow
if x(i,j)>=0 && x(i,j)<position_start_x(1) && y(i,j)>=-(breite/2+margin) && y(i,j)<=(breite/2+margin)                                               %S1
    s=x(i,j);
    t_array(i,j)=y(i,j);
    psi=0;
else if x(i,j)>=position_start_x(1) && x(i,j)<(position_start_x(2)+breite/2+margin) && y(i,j)>=-(breite/2+margin) && y(i,j)<=position_start_y(2)    %S2
        phi=atan((x(i,j)-position_start_x(1))/(position_start_y(2)-y(i,j)));
        r=sqrt((x(i,j)-position_start_x(1))^2 + (position_start_y(2)-y(i,j))^2);
        s=data(1)*phi+s_values(1);
        t_array(i,j)=data(1)-r;
        psi=phi;
        
else if x(i,j)>=(position_start_x(2)-breite/2-margin) && x(i,j)<=(position_start_x(2)+breite/2+margin) && y(i,j)>position_start_y(2) && y(i,j)<position_start_y(3)  %S3
        s=s_values(2)+(y(i,j)-position_start_y(2));
        t_array(i,j)=position_start_x(2)-x(i,j);
        psi=pi/2;
        
else if  x(i,j)<=(position_start_x(3)+breite/2+margin) && x(i,j)>=(position_start_x(4)) && y(i,j)>=position_start_y(3) && y(i,j)<=(position_start_y(4)+breite/2+margin)   %S4
        phi=atan((y(i,j)-position_start_y(3))/(x(i,j)-position_start_x(4)));
        r=sqrt((y(i,j)-position_start_y(3))^2+(x(i,j)-position_start_x(4))^2);
        s=s_values(3)+data(2)*phi;
        t_array(i,j)=data(2)-r;
        psi=pi/2+phi;
        
else if x(i,j)<position_start_x(4) && x(i,j)>position_start_x(5) && y(i,j)>=(position_start_y(4)-breite/2-margin) && y(i,j)<(position_start_y(4)+breite/2+margin)   %S5
        s=s_values(4)+(position_start_x(4)-x(i,j));
        t_array(i,j)=position_start_y(4)-y(i,j);
        psi=pi;
        
else if x(i,j)<=position_start_x(5) && x(i,j)>=(position_start_x(6)-breite/2-margin) && y(i,j)>=position_start_y(6) && y(i,j)<=(position_start_y(5)+breite/2+margin)   %S6
        phi=atan(-x(i,j)/(y(i,j)-position_start_y(6)));
        r=sqrt((x(i,j))^2+(y(i,j)-position_start_y(6))^2);
        s=s_values(5)+data(3)*phi;
        t_array(i,j)=data(3)-r;
        psi=pi+phi;
        
else if x(i,j)>=(position_start_x(6)-breite/2-margin) && x(i,j)<=(position_start_x(6)+breite/2+margin) && y(i,j)>position_start_y(7) && y(i,j)<position_start_y(6)   %S7
        s=s_values(6)+(position_start_y(6)-y(i,j));
        t_array(i,j)=x(i,j)-position_start_x(6);
        psi=3*pi/2;
        
else if x(i,j)>=(position_start_x(7)-breite/2-margin) && x(i,j)<0 && y(i,j)>=(-breite/2-margin) && y(i,j)<=position_start_y(7)   %S8
        phi=atan((position_start_y(7)-y(i,j))/(-x(i,j)));
        r=sqrt((position_start_y(7)-y(i,j))^2+(x(i,j))^2);
        s=s_values(7)+data(4)*phi;
        t_array(i,j)=data(4)-r;
        psi=3*pi/2+phi;     
        

     else
         s=0;
         t_array(i,j)=0;
         psi=0;

    end
    end
    end
    end
    end
    end
    end
end
end
end
t=t_array;    
z=0;
mue=1;

== matlab function ADAS/Sensors_ADAS/Front_Mid_Range_Radar_Sensor/First_STage_Coordinate_Transformation/Radar_Triangles_Transformation_From_Local2Global/Coord_Transformatin_Rotation ==
  data: roll input double; Trans_Local2Global output double; pitch input double; yaw input double
function Trans_Local2Global  = fcn(roll, pitch, yaw)


Trans_Local2Global=[ cos(pitch)*cos(yaw) cos(yaw)*sin(pitch)*sin(roll) - cos(roll)*sin(yaw) sin(roll)*sin(yaw) + cos(roll)*cos(yaw)*sin(pitch);
cos(pitch)*sin(yaw) cos(roll)*cos(yaw) + sin(pitch)*sin(roll)*sin(yaw) cos(roll)*sin(pitch)*sin(yaw) - cos(yaw)*sin(roll);
         -sin(pitch)                               cos(pitch)*sin(roll)                               cos(pitch)*cos(roll)];
